simulink model "testTurningMachine"  (R2025a)
settings: Solver=VariableStepAuto  StartTime=0.0  StopTime=10.0  RelTol=1e-3
libraries: StdLib x11, ProductionLinePLib x1
settings Model: Creator=peter  LastModifiedBy=peter
settings RTWCC: GPUComputeCapability=3.5

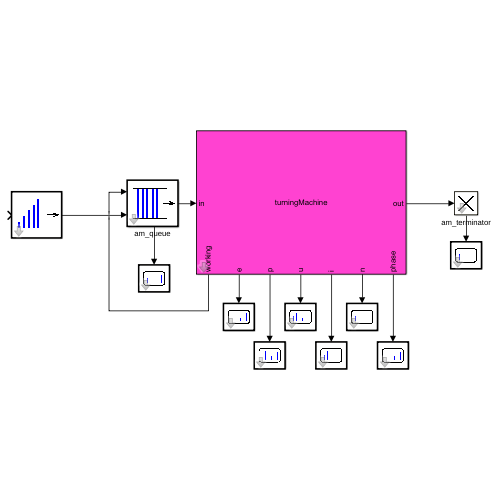
[thumbnail: Simulink's stored preview of the top-level diagram]
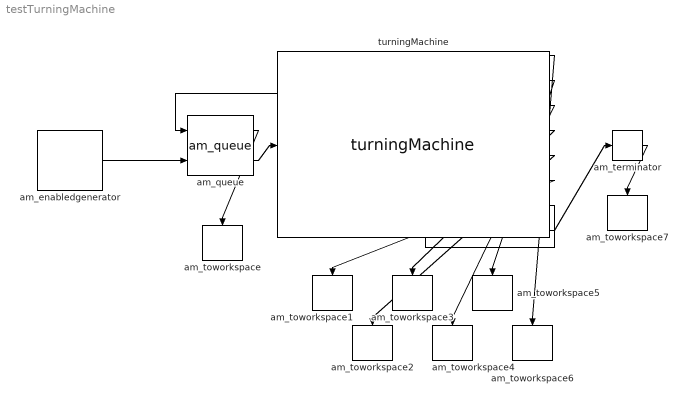
== system testTurningMachine ==
  am_enabledgenerator : StdLib/am_enabledgenerator  tG=3000  n0=0  nG=4  tD=[0,2]  tau=[0,1]  debug=0
  am_queue : StdLib/am_queue  tD=[0,5]  tau=[0,5]  debug=0
  am_terminator : StdLib/am_terminator  tau=[0,1]  debug=0
  am_toworkspace : StdLib/am_toworkspace  varname="\"nq\""  t0=0  format="\"vector\""  tau=[0,5]  debug=0
  am_toworkspace1 : StdLib/am_toworkspace  varname="\"E\""  t0=0  format="\"vector\""  tau=[0,5]  debug=0
  am_toworkspace2 : StdLib/am_toworkspace  varname="\"P\""  t0=0  format="\"vector\""  tau=[0,5]  debug=0
  am_toworkspace3 : StdLib/am_toworkspace  varname="\"u\""  t0=0  format="\"vector\""  tau=[0,5]  debug=0
  am_toworkspace4 : StdLib/am_toworkspace  varname="\"i\""  t0=0  format="\"vector\""  tau=[0,5]  debug=0
  am_toworkspace5 : StdLib/am_toworkspace  varname="\"n\""  t0=0  format="\"vector\""  tau=[0,5]  debug=0
  am_toworkspace6 : StdLib/am_toworkspace  varname="\"phase\""  t0=0  format="\"vector\""  tau=[0,5]  debug=0
  am_toworkspace7 : StdLib/am_toworkspace  varname="\"nout\""  t0=0  format="\"vector\""  tau=[0,5]  debug=0
  turningMachine : ProductionLinePLib/turningMachine  turning_time=20*60  ap_ug=0.5  ap_og=1.5  P_ap=0.6  f_ug=0.1  f_og=0.5  P_f=0.4  vc_ug=150  vc_og=350  P_vc=0.5  ap=0  f=0  vc=0  tauInt=[0,100]  tauCont=[0,100]  tau=[0,1]  debug=0
      settings: LibrarySourceBlock=ProductionLineLib_CM/turning
  wires:
  am_enabledgenerator/1 -> am_queue/1
  turningMachine/1 -> am_terminator/1
  turningMachine/2 -> am_queue/2
  am_queue/1 -> turningMachine/1
  am_queue/2 -> am_toworkspace/1
  am_terminator/1 -> am_toworkspace7/1
  turningMachine/3 -> am_toworkspace1/1
  turningMachine/4 -> am_toworkspace2/1
  turningMachine/5 -> am_toworkspace3/1
  turningMachine/6 -> am_toworkspace4/1
  turningMachine/7 -> am_toworkspace5/1
  turningMachine/8 -> am_toworkspace6/1
